simulink model "AutoCart"  (R2022a)
settings: Solver=FixedStepAuto  StartTime=0.0  StopTime=inf  RelTol=1e-3
undefined symbols (not defined in the file): GO, RemoteControllerApp5, Reverse, Set_Speed, Speed_display, Steer
libraries: androiduilib x9, androidcommunicationlib x2
settings Model: Creator=Admin  LastModifiedBy=Amro
settings OptimizationCC: EnhancedBackFolding=on  PassReuseOutputArgsAs=Individual arguments  ZeroExternalMemoryAtStartup=off  ZeroInternalMemoryAtStartup=off  MaxStackSize=64  OptimizeBlockOrder=speed  DifferentSizesBufferReuse=on  OptimizationCustomize=off  EfficientTunableParamExpr=on
settings DebuggingCC: ParameterTunabilityLossMsg=error  UnconnectedInputMsg=warning  UnconnectedOutputMsg=warning  UnconnectedLineMsg=warning
settings HardwareCC: ProdBitPerPointer=32  ProdBitPerSizeT=32  ProdBitPerPtrDiffT=32  ProdLargestAtomicInteger=Long  ProdLargestAtomicFloat=Double  ProdWordSize=32  ProdHWDeviceType=ARM Compatible->ARM Cortex
settings SFSimCC: MATLABDynamicMemAlloc=off
settings RTWCC: SystemTargetFile=ert.tlc  HardwareBoard=Android Device  TLCOptions="-aInlineSetEventsForThisBaseRateFcn=TLC_FALSE -aSuppressMultiTaskScheduler=TLC_FALSE  -aRateBasedStepFcn=0"  TemplateMakefile=ert_default_tmf  RTWVerbose=off  Toolchain=Android SDK/NDK Tools  DLArmComputeVersion=19.05
settings CodeAppCC: ForceParamTrailComments=on  IgnoreCustomStorageClasses=off  OperatorAnnotations=on  SimulinkDataObjDesc=on  SFDataObjDesc=on  InsertBlockDesc=on
settings ERTTargetCC: SupportVariableSizeSignals=on

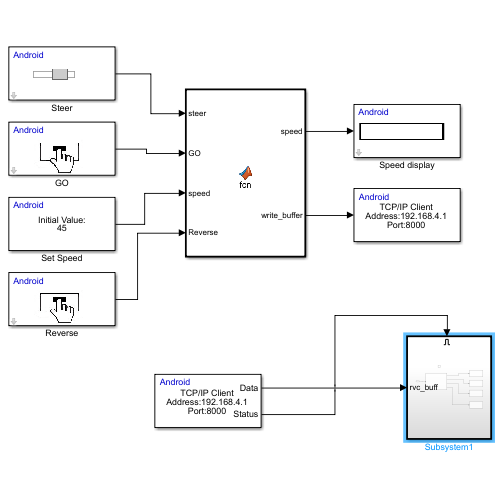
[thumbnail: Simulink's stored preview of the top-level diagram]
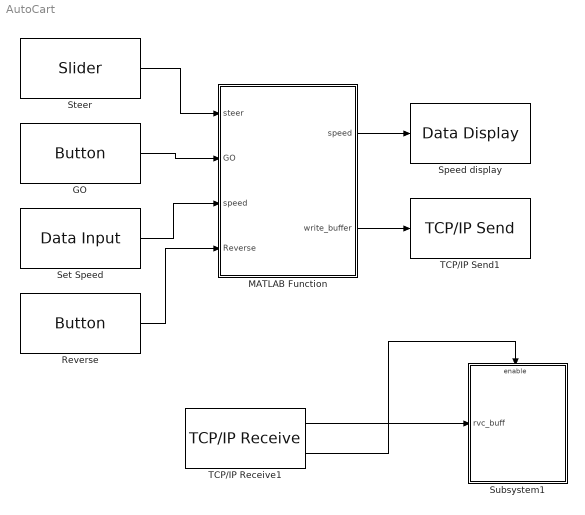
== system AutoCart ==
  GO : androiduilib/Button  ButtonState=Not pressed  ButtonId=RemoteControllerApp5/GO  State=off  SampleTime=0.1  BlockPlatform=Android
      settings: SourceProductBaseCode=ANDROID
  MATLAB Function : MATLAB Function  TreatAsAtomicUnit=on
  Reverse : androiduilib/Button  ButtonState=Not pressed  ButtonId=RemoteControllerApp5/Reverse  State=off  SampleTime=0.1  BlockPlatform=Android
      settings: SourceProductBaseCode=ANDROID
  Set Speed : androiduilib/Data Input  isCharVector=off  Value=45  CharVector=Hello World  OutputDataType=single  maxCharVectorSize=100  DataInputId=RemoteControllerApp5/Set_Speed  SampleTime=0.1
      settings: SourceProductBaseCode=ANDROID
  Speed display : androiduilib/Data Display  DataDisplayId=RemoteControllerApp5/Speed_display  Format=Float  Precision=6  SimulateUsing=Code generation  blockPlatform=Android
      settings: SourceProductBaseCode=ANDROID
  Steer : androiduilib/Slider  Min=-60  Value=0  Max=60  Resolution=5  SliderId=RemoteControllerApp5/Steer  SampleTime=0.1  BlockPlatform=Android
      settings: SourceProductBaseCode=ANDROID
  Subsystem1 : Subsystem
  TCP/IP Receive1 : androidcommunicationlib/TCP//IP Receive  TCPReceiveId=RemoteControllerApp5/TCP//IP_Receive1  Mode_=Client  LocalServerPort_=25000  RemoteAddr_=192.168.4.1  RemoteServerPort_=8000  DataType_=uint8  DataSize_=22  SampleTime_=0.1  ClientPortBindingSelection_=off  ClientPortToBind_=35000  BlockingMode_=off  BlockTimeout_=0.1
      settings: SourceProductBaseCode=ANDROID
  TCP/IP Send1 : androidcommunicationlib/TCP//IP Send  TCPSendId=RemoteControllerApp5/TCP//IP_Send1  Mode_=Client  LocalServerPort_=25000  RemoteAddr_=192.168.4.1  RemoteServerPort_=8000  ClientPortBindingSelection_=off  ClientPortToBind_=35000  BlockingMode_=off  BlockTimeout_=0.1
      settings: SourceProductBaseCode=ANDROID
  wires:
  MATLAB Function/2(write_buffer) -> TCP/IP Send1/1
  TCP/IP Receive1/1 -> Subsystem1/1(rvc_buff)
  TCP/IP Receive1/2 -> Subsystem1/Enable
  Steer/1 -> MATLAB Function/1(steer)
  GO/1 -> MATLAB Function/2(GO)
  MATLAB Function/1(speed) -> Speed display/1
  Set Speed/1 -> MATLAB Function/3("speed ")
  Reverse/1 -> MATLAB Function/4(Reverse)

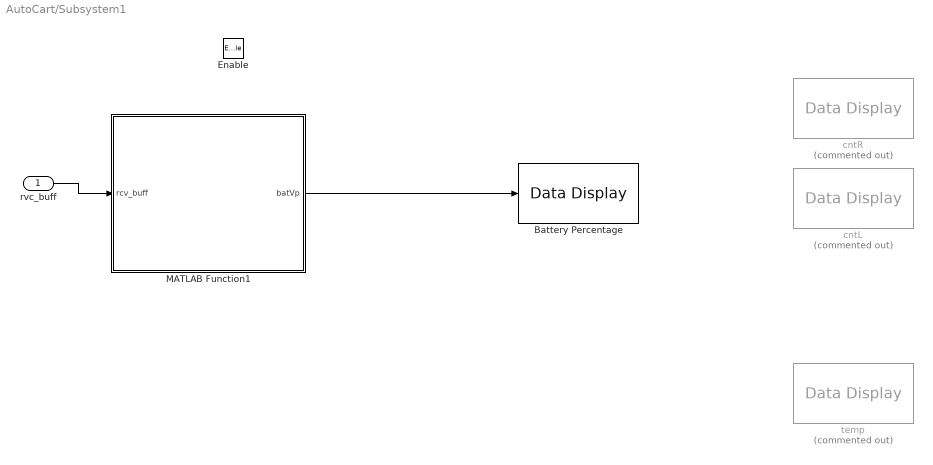
== system AutoCart/Subsystem1 ==
  rvc_buff : Inport
  Enable : EnablePort
  Battery Percentage : androiduilib/Data Display  DataDisplayId=RemoteControllerApp5/Subsystem1/Battery_Percentage  Format=Float  Precision=6  SimulateUsing=Code generation  blockPlatform=Android
      settings: SourceProductBaseCode=ANDROID
  MATLAB Function1 : MATLAB Function  TreatAsAtomicUnit=on
  cntL : androiduilib/Data Display  Commented=on  DataDisplayId=RemoteControllerApp3/Subsystem1/cntL  Format=Float  Precision=6  SimulateUsing=Code generation  blockPlatform=Android
      settings: SourceProductBaseCode=ANDROID
  cntR : androiduilib/Data Display  Commented=on  DataDisplayId=RemoteControllerApp3/Subsystem1/cntR  Format=Float  Precision=6  SimulateUsing=Code generation  blockPlatform=Android
      settings: SourceProductBaseCode=ANDROID
  temp : androiduilib/Data Display  Commented=on  DataDisplayId=RemoteControllerApp3/Subsystem1/temp  Format=Float  Precision=6  SimulateUsing=Code generation  blockPlatform=Android
      settings: SourceProductBaseCode=ANDROID
  wires:
  rvc_buff/1 -> MATLAB Function1/1(rcv_buff)
  MATLAB Function1/1(batVp) -> Battery Percentage/1

== matlab function AutoCart/Subsystem1/MATLAB Function1 ==
  data: rcv_buff input; batVp output single size=1
function batVp  = fcn(rcv_buff)
% header = rvc_buff(1:2);
% cmd1 = rvc_buff(3:4);
% cmd2 = rvc_buff(5:6);
% spdR = rvc_buff(7:8);
% spdL = rvc_buff(9:10);
% temp = rvc_buff(17:18);
% cmdLED = rvc_buff(19:20);
% chkSum = rvc_buff(21:22);
% 
cntR = typecast(rcv_buff(11:12) , 'int16');
cntL = typecast(rcv_buff(13:14) , 'int16');
batV = single(typecast(rcv_buff(15:16) , 'int16'))/100;
batVp = ((batV - 36)*100 / (41-36));
temp = single(typecast(rcv_buff(17:18) , 'int16'))/100;

== matlab function AutoCart/MATLAB Function ==
  data: speed output; write_buffer output size=[1 8]; steer input single size=1; GO input boolean size=1; speed input single; Reverse input
function [speed, write_buffer] = fcn(steer, GO, speed, Reverse)



        


if (GO == false && Reverse == false)
    speed = single(0);
    steer = single(0);

    
end

if (Reverse)
        speed = -1*speed;
        
end

if(speed<0)
    speed = speed + 65536;
end
if(steer<0)
    steer = steer + 65536;
end





start = uint16(43981);
steerp = uint16(steer);
speedp = uint16(speed);
chkSum = bitxor(bitxor(start,steerp),speedp);
chkSum = typecast((chkSum),'uint16');
write_buffer = [typecast((start),'uint8'),typecast((steerp),'uint8'),typecast((speedp),'uint8'),typecast((chkSum),'uint8')];
